simulink model "example_madgwick"  (R2016a)
settings: Solver=VariableStepAuto  StartTime=0.0  StopTime=60  RelTol=1e-3
values from neighbouring files (symbols this model uses):
  omega_max_lim = 2500    [init.m]
  omega_min_lim = 0    [init.m]
  T_max_lim = Tp - (Tp - Tm) * sat_lim    [init.m]
  tau_max_lim = 1e-5    (= 1e-05)    [init.m]
  tau_min_lim = -1e-5    (= -1e-05)    [init.m]
undefined symbols (not defined in the file or in its folder): inner_h
settings Model: Creator=mgreiff  LastModifiedBy=mgreiff

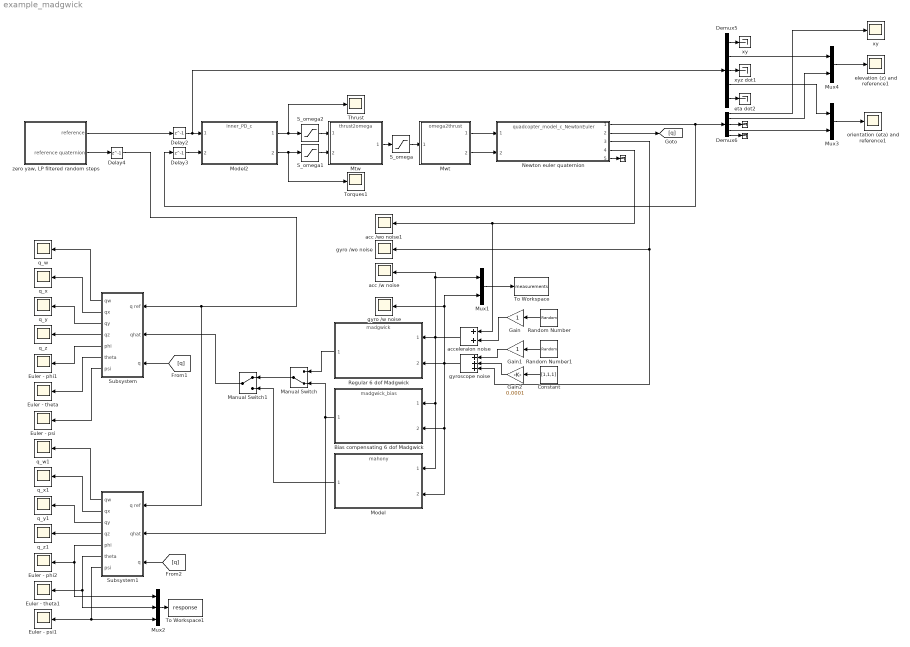
== system example_madgwick ==
  "            " : Terminator
  "              " : Terminator
  "               " : Terminator
  "   eta dot2" : Terminator
  "   xy" : Terminator
  "  xyz dot1" : Terminator
  Bias compensating 6 dof Madgwick : ModelReference  ModelNameDialog=madgwick_bias.slx  SimulationMode=Normal  ModelReferenceVersion=1.26
  Constant : Constant  Value=[1,1,1]
  Delay2 : Delay  DelayLength=1  InitialCondition=0  SampleTime=inner_h
  Delay3 : Delay  DelayLength=1  InitialCondition=0  SampleTime=inner_h
  Delay4 : Delay  DelayLength=1  InitialCondition=0  SampleTime=inner_h
  Demux5 : Demux  Outputs=[2,1,3,3,3]
  Demux6 : Demux  Outputs=[2,1,3,3,3]
  Euler - phi1 : Scope
  Euler - phi2 : Scope
  Euler - psi : Scope
  Euler - psi1 : Scope
  Euler - theta : Scope
  Euler - theta1 : Scope
  Gain : Gain
  Gain1 : Gain
  Gain2 : Gain  Gain=0.0001
  Manual Switch : ManualSwitch  CurrentSetting=0
  Manual Switch1 : ManualSwitch
  Model : ModelReference  ModelNameDialog=mahony.slx  SimulationMode=Normal  ModelReferenceVersion=1.2
  Model2 : ModelReference  ModelNameDialog=inner_PD_c.mdl  SimulationMode=Normal  ModelReferenceVersion=1.87
  Mtw : ModelReference  ModelNameDialog=thrust2omega.mdl  SimulationMode=Normal  ModelReferenceVersion=1.3
  Mux1 : Mux  Inputs=2
  Mux2 : Mux  Inputs=3
  Mux3 : Mux  Inputs=2
  Mux4 : Mux  Inputs=2
  Mwt : ModelReference  ModelNameDialog=omega2thrust.mdl  SimulationMode=Normal  ModelReferenceVersion=1.3
  Newton euler quaternion : ModelReference  ModelNameDialog=quadcopter_model_c_NewtonEuler.mdl  SimulationMode=Normal  ModelReferenceVersion=1.325
  Random Number : RandomNumber  Mean=[0,0,0]  Variance=[0.5, 0.5, 0.5].^2
  Random Number1 : RandomNumber  Mean=[0,0,0]  Variance=[0.05,0.05,0.05].^2
  Regular 6 dof Madgwick : ModelReference  ModelNameDialog=madgwick.slx  SimulationMode=Normal  ModelReferenceVersion=1.26
  S_omega : Saturate  UpperLimit=omega_max_lim  LowerLimit=omega_min_lim
  S_omega1 : Saturate  UpperLimit=tau_max_lim  LowerLimit=tau_min_lim
  S_omega2 : Saturate  UpperLimit=T_max_lim  LowerLimit=tau_min_lim
  Subsystem : Subsystem
  Subsystem1 : Subsystem
  Thrust : Scope
  To Workspace : ToWorkspace  VariableName=measurements  SaveFormat=Timeseries  SampleTime=-1
  To Workspace1 : ToWorkspace  VariableName=response  SaveFormat=Timeseries  SampleTime=-1
  Torques1 : Scope
  acc /w noise : Scope
  acc /wo noise1 : Scope
  acceleraion noise : Sum
  elevation (z) and reference1 : Scope
  gyro /w noise : Scope
  gyro /wo noise : Scope
  gyroscope noise : Sum  Inputs=+++
  orientation (eta) and reference1 : Scope
  q_w : Scope
  q_w1 : Scope
  q_x : Scope
  q_x1 : Scope
  q_y : Scope
  q_y1 : Scope
  q_z : Scope
  q_z1 : Scope
  xy : Scope
  "zero yaw, LP filtered random steps" : Subsystem
  wires:
  Demux5/2 -> Mux4/1
  Mux4/1 -> elevation (z) and reference1/1
  Mux3/1 -> orientation (eta) and reference1/1
  Demux5/3 -> "  xyz dot1"/1
  Demux5/5 -> "   eta dot2"/1
  Demux5/1 -> "   xy"/1
  Demux5/4 -> Mux3/1
  Delay2/1 -> Model2/1, Demux5/1
  Demux6/2 -> Mux4/2
  Demux6/1 -> xy/1
  "zero yaw, LP filtered random steps"/1(reference) -> Delay2/1
  Mtw/1 -> S_omega/1
  Mwt/1 -> Newton euler quaternion/1
  S_omega/1 -> Mwt/1
  Model2/2 -> S_omega1/1, Torques1/1
  Model2/1 -> S_omega2/1, Thrust/1
  Delay3/1 -> Model2/2
  S_omega1/1 -> Mtw/2
  S_omega2/1 -> Mtw/1
  acceleraion noise/1 -> acc /w noise/1, Mux1/1, Model/1, Bias compensating 6 dof Madgwick/1, Regular 6 dof Madgwick/1
  gyroscope noise/1 -> Regular 6 dof Madgwick/2, Mux1/2, gyro /w noise/1, Model/2, Bias compensating 6 dof Madgwick/2
  Random Number/1 -> Gain/1
  Random Number1/1 -> Gain1/1
  Gain/1 -> acceleraion noise/2
  Gain1/1 -> gyroscope noise/1
  Subsystem/1(qw) -> q_w/1
  Subsystem/2(qx) -> q_x/1
  Subsystem/3(qy) -> q_y/1
  Subsystem/4(qz) -> q_z/1
  Subsystem/5(phi) -> Euler - phi1/1
  Subsystem/6(theta) -> Euler - theta/1
  Subsystem/7(psi) -> Euler - psi/1
  [q] -> Subsystem/3(q)
  "zero yaw, LP filtered random steps"/2(reference quaternion) -> Delay4/1
  Delay4/1 -> Subsystem1/1(q ref), Subsystem/1(q ref)
  Mwt/2 -> Newton euler quaternion/2
  Newton euler quaternion/4 -> acceleraion noise/1, acc /wo noise1/1
  Newton euler quaternion/5 -> "            "/1
  Newton euler quaternion/3 -> gyroscope noise/3, gyro /wo noise/1
  Newton euler quaternion/1 -> Delay3/1, Demux6/1
  Newton euler quaternion/2 -> [q]
  Demux6/3 -> "              "/1
  Demux6/5 -> "               "/1
  Demux6/4 -> Mux3/2
  Regular 6 dof Madgwick/1 -> Manual Switch/1
  Bias compensating 6 dof Madgwick/1 -> Manual Switch/2, Subsystem1/2(qhat)
  Manual Switch/1 -> Manual Switch1/1
  Manual Switch1/1 -> Subsystem/2(qhat)
  Model/1 -> Manual Switch1/2
  Subsystem1/1(qw) -> q_w1/1
  Subsystem1/2(qx) -> q_x1/1
  Subsystem1/3(qy) -> q_y1/1
  Subsystem1/4(qz) -> q_z1/1
  Subsystem1/5(phi) -> Mux2/1, Euler - phi2/1
  Subsystem1/6(theta) -> Mux2/2, Euler - theta1/1
  Subsystem1/7(psi) -> Mux2/3, Euler - psi1/1
  [q] -> Subsystem1/3(q)
  Constant/1 -> Gain2/1
  Gain2/1 -> gyroscope noise/2
  Mux1/1 -> To Workspace/1
  Mux2/1 -> To Workspace1/1

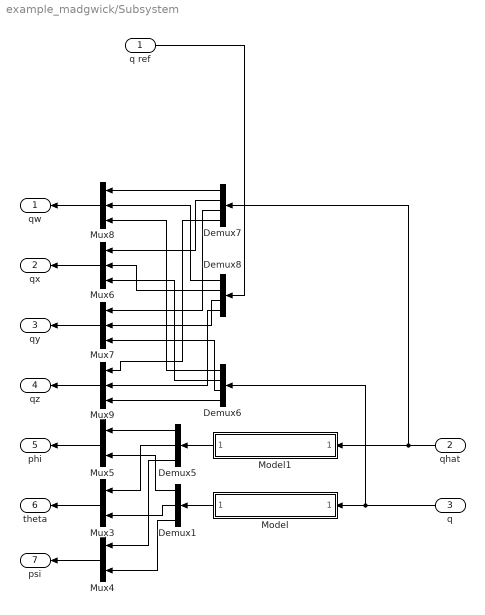
== system example_madgwick/Subsystem ==
  q ref : Inport
  qhat : Inport  Port=2
  q : Inport  Port=3
  Demux1 : Demux  Outputs=3
  Demux5 : Demux  Outputs=3
  Demux6 : Demux
  Demux7 : Demux
  Demux8 : Demux
  Model : ModelReference  ModelNameDialog=quaternion2euler.mdl  SimulationMode=Normal  ModelReferenceVersion=1.92
  Model1 : ModelReference  ModelNameDialog=quaternion2euler.mdl  SimulationMode=Normal  ModelReferenceVersion=1.92
  Mux3 : Mux  Inputs=2
  Mux4 : Mux  Inputs=2
  Mux5 : Mux  Inputs=2
  Mux{6..9} (4 alike) : Mux  Inputs=3
  qw : Outport
  qx : Outport  Port=2
  qy : Outport  Port=3
  qz : Outport  Port=4
  phi : Outport  Port=5
  theta : Outport  Port=6
  psi : Outport  Port=7
  wires:
  Demux6/2 -> Mux6/3
  Mux5/1 -> phi/1
  Demux8/3 -> Mux7/2
  Demux7/4 -> Mux9/1
  Mux9/1 -> qz/1
  Mux7/1 -> qy/1
  Mux6/1 -> qx/1
  Demux6/1 -> Mux8/3
  Mux4/1 -> psi/1
  Mux3/1 -> theta/1
  Model1/1 -> Demux5/1
  qhat/1 -> Model1/1, Demux7/1
  Demux7/2 -> Mux6/1
  Demux7/1 -> Mux8/1
  Demux6/4 -> Mux9/3
  Demux8/4 -> Mux9/2
  Demux8/2 -> Mux6/2
  Demux6/3 -> Mux7/3
  Mux8/1 -> qw/1
  q ref/1 -> Demux8/1
  Demux7/3 -> Mux7/1
  Demux8/1 -> Mux8/2
  Model/1 -> Demux1/1
  q/1 -> Demux6/1, Model/1
  Demux5/1 -> Mux5/1
  Demux5/2 -> Mux3/1
  Demux5/3 -> Mux4/1
  Demux1/3 -> Mux4/2
  Demux1/2 -> Mux3/2
  Demux1/1 -> Mux5/2

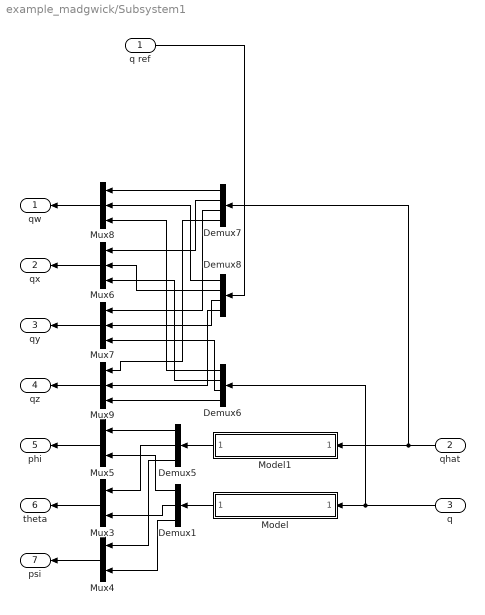
== system example_madgwick/Subsystem1 ==
  q ref : Inport
  qhat : Inport  Port=2
  q : Inport  Port=3
  Demux1 : Demux  Outputs=3
  Demux5 : Demux  Outputs=3
  Demux6 : Demux
  Demux7 : Demux
  Demux8 : Demux
  Model : ModelReference  ModelNameDialog=quaternion2euler.mdl  SimulationMode=Normal  ModelReferenceVersion=1.92
  Model1 : ModelReference  ModelNameDialog=quaternion2euler.mdl  SimulationMode=Normal  ModelReferenceVersion=1.92
  Mux3 : Mux  Inputs=2
  Mux4 : Mux  Inputs=2
  Mux5 : Mux  Inputs=2
  Mux{6..9} (4 alike) : Mux  Inputs=3
  qw : Outport
  qx : Outport  Port=2
  qy : Outport  Port=3
  qz : Outport  Port=4
  phi : Outport  Port=5
  theta : Outport  Port=6
  psi : Outport  Port=7
  wires:
  Demux6/2 -> Mux6/3
  Mux5/1 -> phi/1
  Demux8/3 -> Mux7/2
  Demux7/4 -> Mux9/1
  Mux9/1 -> qz/1
  Mux7/1 -> qy/1
  Mux6/1 -> qx/1
  Demux6/1 -> Mux8/3
  Mux4/1 -> psi/1
  Mux3/1 -> theta/1
  Model1/1 -> Demux5/1
  qhat/1 -> Model1/1, Demux7/1
  Demux7/2 -> Mux6/1
  Demux7/1 -> Mux8/1
  Demux6/4 -> Mux9/3
  Demux8/4 -> Mux9/2
  Demux8/2 -> Mux6/2
  Demux6/3 -> Mux7/3
  Mux8/1 -> qw/1
  q ref/1 -> Demux8/1
  Demux7/3 -> Mux7/1
  Demux8/1 -> Mux8/2
  Model/1 -> Demux1/1
  q/1 -> Demux6/1, Model/1
  Demux5/1 -> Mux5/1
  Demux5/2 -> Mux3/1
  Demux5/3 -> Mux4/1
  Demux1/3 -> Mux4/2
  Demux1/2 -> Mux3/2
  Demux1/1 -> Mux5/2

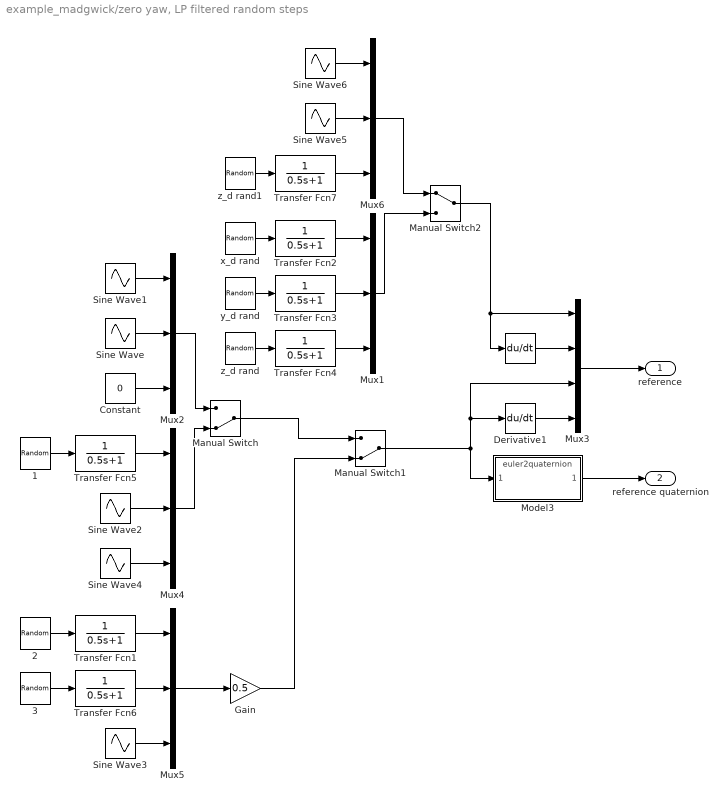
== system example_madgwick/zero yaw, LP filtered random steps ==
  "        " : Derivative
  "   1" : UniformRandomNumber  Minimum=-0.2  Maximum=0.2  Seed=5  SampleTime=5
  "   2" : UniformRandomNumber  Seed=5  SampleTime=5
  "   3" : UniformRandomNumber  Seed=3  SampleTime=5
  Constant : Constant  Value=0
  Derivative1 : Derivative
  Gain : Gain  Gain=0.5
  Manual Switch : ManualSwitch  CurrentSetting=0
  Manual Switch1 : ManualSwitch  CurrentSetting=0
  Manual Switch2 : ManualSwitch
  Model3 : ModelReference  ModelNameDialog=euler2quaternion.mdl  SimulationMode=Normal  ModelReferenceVersion=1.5
  Mux{1..2,4..6} (5 alike) : Mux  Inputs=3
  Mux3 : Mux  Inputs=[3,3,3,3]
  Sine Wave : Sin  Amplitude=0.4  SampleTime=0
  Sine Wave1 : Sin  Amplitude=0.4  Phase=60  SampleTime=0
  Sine Wave2 : Sin  Amplitude=0.1  SampleTime=0
  Sine Wave3 : Sin  Amplitude=2  Frequency=0.5  SampleTime=0
  Sine Wave4 : Sin  Amplitude=0.1  SampleTime=0
  Sine Wave5 : Sin  Amplitude=0.1  SampleTime=0
  Sine Wave6 : Sin  Amplitude=0.1  Phase=60  SampleTime=0
  Transfer Fcn{1..7} (7 alike) : TransferFcn  Denominator=[0.5 1]
  x_d rand : UniformRandomNumber  Minimum=-30  Maximum=30  SampleTime=10
  y_d rand : UniformRandomNumber  Minimum=-30  Maximum=30  Seed=1  SampleTime=10
  z_d rand : UniformRandomNumber  Minimum=0  Maximum=2  Seed=2  SampleTime=5
  z_d rand1 : UniformRandomNumber  Minimum=0  Seed=2  SampleTime=10
  reference : Outport
  reference quaternion : Outport  Port=2
  wires:
  Mux3/1 -> reference/1
  Derivative1/1 -> Mux3/4
  "        "/1 -> Mux3/2
  Sine Wave1/1 -> Mux2/1
  Sine Wave/1 -> Mux2/2
  Constant/1 -> Mux2/3
  x_d rand/1 -> Transfer Fcn2/1
  y_d rand/1 -> Transfer Fcn3/1
  z_d rand/1 -> Transfer Fcn4/1
  Transfer Fcn2/1 -> Mux1/1
  Transfer Fcn3/1 -> Mux1/2
  Transfer Fcn4/1 -> Mux1/3
  "   1"/1 -> Transfer Fcn5/1
  Transfer Fcn5/1 -> Mux4/1
  Sine Wave2/1 -> Mux4/2
  Sine Wave4/1 -> Mux4/3
  Mux2/1 -> Manual Switch/1
  Mux4/1 -> Manual Switch/2
  "   2"/1 -> Transfer Fcn1/1
  Transfer Fcn1/1 -> Mux5/1
  Transfer Fcn6/1 -> Mux5/2
  Sine Wave3/1 -> Mux5/3
  Mux5/1 -> Gain/1
  Manual Switch/1 -> Manual Switch1/1
  Manual Switch1/1 -> Mux3/3, Derivative1/1, Model3/1
  "   3"/1 -> Transfer Fcn6/1
  Model3/1 -> reference quaternion/1
  Gain/1 -> Manual Switch1/2
  Sine Wave6/1 -> Mux6/1
  Sine Wave5/1 -> Mux6/2
  Transfer Fcn7/1 -> Mux6/3
  Mux6/1 -> Manual Switch2/1
  Mux1/1 -> Manual Switch2/2
  Manual Switch2/1 -> Mux3/1, "        "/1
  z_d rand1/1 -> Transfer Fcn7/1
